simulink model "Problema4_1"  (R2018a)
settings: Solver=ode23tb  StartTime=0.0  StopTime=.1  RelTol=1e-8  EnableMultiTasking=on
libraries: powerlib x17
settings Model: Creator=Moni  LastModifiedBy=Valen
settings SolverCC: SolverResetMethod=Robust
settings DataIOCC: SaveFormat=Array
settings OptimizationCC: LifeSpan=inf
settings DebuggingCC: SolverPrmCheckMsg=warning  SFUnexpectedBacktrackingDiag=warning  SFNoUnconditionalDefaultTransitionDiag=warning  SFExecutionAtInitializationDiag=none
settings HardwareCC: ProdBitPerPointer=32  ProdBitPerSizeT=32  ProdBitPerPtrDiffT=32  ProdLargestAtomicFloat=None  ProdIntDivRoundTo=Undefined  ProdEndianess=Unspecified  ProdWordSize=32  ProdHWDeviceType=32-bit Generic
settings ModelReferenceCC: PropagateSignalLabelsOutOfModel=off
settings CodeAppCC: StateflowObjectComments=on
settings GRTTargetCC: TargetLangStandard=C89/C90 (ANSI)  GeneratePreprocessorConditionals=Disable all
settings ConfigComp: CovMetricSettings=dw  CovHtmlReporting=on  CovSaveCumulativeToWorkspaceVar=on  CovSaveSingleToWorkspaceVar=on  CovExternalEMLEnable=off  CovSFcnEnable=off
settings SimscapeCC: SimscapeNormalizeSystem=off

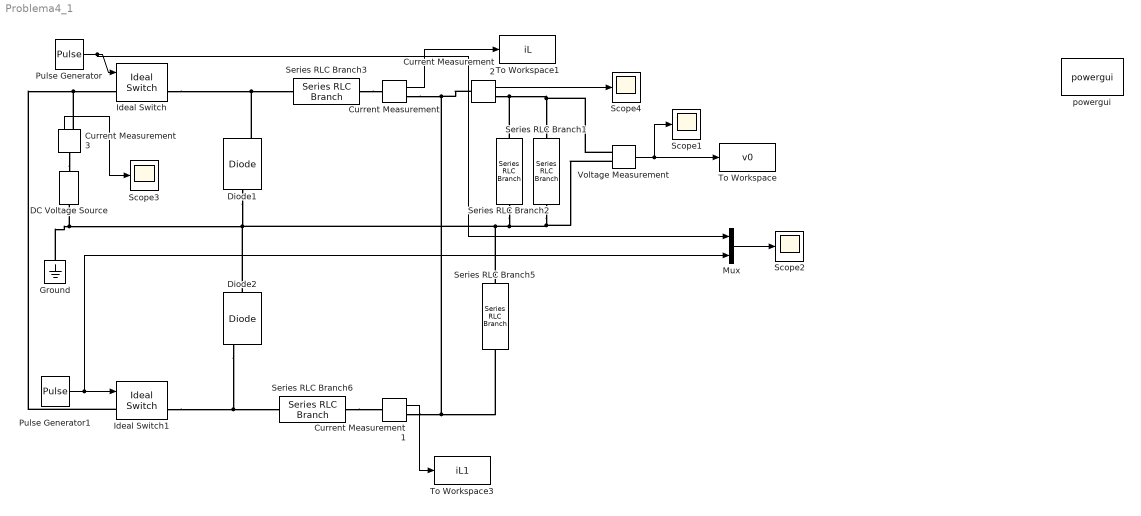
== system Problema4_1 ==
  Current Measurement{,1..3} (4 alike) : powerlib/Measurements/Current Measurement  PhasorSimulation=off  OutputType=Complex  PSBequivalent=0
  DC Voltage Source : powerlib/Electrical Sources/DC Voltage Source  Amplitude=30  Measurements=None
  Diode1 : powerlib/Power Electronics/Diode  Ron=0.001  Lon=0  Vf=0  IC=0  UseSnubber=off  Rs=500  Cs=250e-9  Measurements=on
  Diode2 : powerlib/Power Electronics/Diode  Ron=0.001  Lon=0  Vf=0  IC=0  UseSnubber=off  Rs=500  Cs=250e-9  Measurements=on
  Ground : powerlib/Elements/Ground  LConnTagsString=a
  Ideal Switch : powerlib/Power Electronics/Ideal Switch  Ron=.00000001  Lon=0  IC=0  Rs=1e5  Cs=inf  Measurements=on
  Ideal Switch1 : powerlib/Power Electronics/Ideal Switch  Ron=.0000001  Lon=0  IC=0  Rs=1e5  Cs=inf  Measurements=on
  Mux : Mux  Inputs=2
  Pulse Generator : DiscretePulseGenerator  PulseType=Time based  Period=4e-6  PulseWidth=26.6667
  Pulse Generator1 : DiscretePulseGenerator  PulseType=Time based  Period=4e-6  PulseWidth=26.6667  PhaseDelay=2e-6
  Scope{1..4} (4 alike) : Scope
  Series RLC Branch1 : powerlib/Elements/Series RLC Branch  LConnTagsString=__new0  RConnTagsString=__new0  BranchType=R  Resistance=.5  Inductance=0  SetiL0=off  InitialCurrent=0  Capacitance=0  Setx0=off  InitialVoltage=0  Measurements=None
  Series RLC Branch2 : powerlib/Elements/Series RLC Branch  LConnTagsString=__new0  RConnTagsString=__new0  BranchType=C  Resistance=.001  Inductance=50e-6  SetiL0=off  InitialCurrent=0  Capacitance=11e-6  Setx0=off  InitialVoltage=0  Measurements=Branch current
  Series RLC Branch3 : powerlib/Elements/Series RLC Branch  LConnTagsString=__new0  RConnTagsString=__new0  BranchType=L  Resistance=.001  Inductance=38.8e-6  SetiL0=off  InitialCurrent=0  Capacitance=1.0  Setx0=off  InitialVoltage=0  Measurements=Branch current
  Series RLC Branch5 : powerlib/Elements/Series RLC Branch  LConnTagsString=__new0  RConnTagsString=__new0  BranchType=C  Resistance=.001  Inductance=50e-6  SetiL0=off  InitialCurrent=0  Capacitance=11e-6  Setx0=off  InitialVoltage=0  Measurements=None
  Series RLC Branch6 : powerlib/Elements/Series RLC Branch  LConnTagsString=__new0  RConnTagsString=__new0  BranchType=L  Resistance=.001  Inductance=38.8e-6  SetiL0=off  InitialCurrent=0  Capacitance=1.0  Setx0=off  InitialVoltage=0  Measurements=Branch current
  To Workspace : ToWorkspace  VariableName=v0  SampleTime=-1
  To Workspace1 : ToWorkspace  VariableName=iL  SampleTime=-1
  To Workspace3 : ToWorkspace  VariableName=iL1  SampleTime=-1
  Voltage Measurement : powerlib/Measurements/Voltage Measurement  PhasorSimulation=off  OutputType=Complex  PSBequivalent=0
  powergui : powerlib/powergui  Priority=1  SimulationMode=Continuous  SampleTime=50e-6  frequency=60  Iterations=50  frequencyindice=0  Pbase=100e6  ErrMax=1e-4  UnitsV=kV  UnitsW=MW  buscounter=0  FunctionMessages=off  echomessages=off  EnableUseOfTLC=off  CurrentSourceSwitches=on  DisableSnubberDevices=off  DisableRonSwitches=off  DisableVfSwitches=off  DisplayEquations=off  SolverType=Tustin  Interpol=off  ExternalGateDelay=off  methode=off  Ts=0  x0status=blocks  SPID=off  SwTol=0  HookPort=off  RestoreLinks=warning  ResistiveCurrentMeasurement=off  Frange=[0:2:500]  Ylog=off  Xlog=on  ShowGrid=off  save=off  variable=ZData  structure=0  ZoomFFT=off  StartTime=0.0  cycles=1  DisplayStyle=1  fundamental=60  FreqAxis=off  MaxFrequency=1000  frequencyindicesteady=1  RmsSteady=1  display=off
  wires:
  Current Measurement/1 -> To Workspace1/1
  Voltage Measurement/1 -> To Workspace/1, Scope1/1
  Pulse Generator/1 -> Mux/1, Ideal Switch/1
  Current Measurement1/1 -> To Workspace3/1
  Pulse Generator1/1 -> Mux/2, Ideal Switch1/1
  Mux/1 -> Scope2/1
  Current Measurement2/1 -> Scope4/1
  Current Measurement3/1 -> Scope3/1
  connections:
  Ground/LConn1 -- Series RLC Branch2/LConn1 -- Voltage Measurement/LConn2 -- Series RLC Branch1/RConn1 -- Series RLC Branch5/LConn1 -- Diode1/LConn1 -- Diode2/LConn1 -- DC Voltage Source/LConn1
  Ideal Switch1/LConn1 -- Current Measurement3/RConn1 -- Ideal Switch/LConn1
  Ideal Switch/RConn1 -- Diode1/RConn1 -- Series RLC Branch3/RConn1
  Series RLC Branch3/LConn1 -- Current Measurement/LConn1
  Current Measurement1/RConn1 -- Series RLC Branch5/RConn1 -- Current Measurement2/LConn1 -- Current Measurement/RConn1
  Diode2/RConn1 -- Ideal Switch1/RConn1 -- Series RLC Branch6/RConn1
  Series RLC Branch6/LConn1 -- Current Measurement1/LConn1
  Voltage Measurement/LConn1 -- Series RLC Branch2/RConn1 -- Current Measurement2/RConn1 -- Series RLC Branch1/LConn1
  Current Measurement3/LConn1 -- DC Voltage Source/RConn1
